simulink model "hydraulic_actuator"  (R2018a)
settings: Solver=ode23t  StartTime=0.0  StopTime=10.0  MaxStep=0.001  RelTol=1e-6  EnableMultiTasking=on
libraries: fl_lib x12, sh_lib x9, nesl_utility x4, simulink x1
Description:
  | Closed-Loop Electrohydraulic Actuator with Proportional Valve
  | 
  | This example shows an actuator that consists of a proportional 4-way directional valve
  | driving a double-acting hydraulic cylinder. The cylinder drives a load consisting of a mass,
  | viscous and Coulomb friction, constant force, and a spring. The actuator is powered
  | by a variable-displacement, pressure-compensated pump, driven by a constant velocity
  | motor. Pipelines between the valve, cylinder, pump, and the tank are simulated
  | with the Hydraulic Pipeline blocks.
  | 
  | 
  | Copyright 2008-2013 The MathWorks, Inc.
settings Model: ExtModeAutoUpdateStatusClock=off  Creator=MathWorks  LastModifiedBy=bpotter
settings DataIOCC: LimitDataPoints=on  SaveFormat=Array  SaveOutput=off  SignalLogging=off  DSMLogging=off  SaveTime=off
settings OptimizationCC: DefaultParameterBehavior=Inlined  ExpressionDepthLimit=2147483647  InitFltsAndDblsToZero=on  LifeSpan=inf
settings DebuggingCC: SaveWithParameterizedLinksMsg=none  SignalResolutionControl=TryResolveAllWithWarning  SolverPrmCheckMsg=warning  MultiTaskDSMMsg=warning  AllowSymbolicDim=off  StateNameClashWarn=warning  StrictBusMsg=ErrorOnBusTreatedAsVector  NonBusSignalsTreatedAsBus=error  SFUnexpectedBacktrackingDiag=warning  SFNoUnconditionalDefaultTransitionDiag=warning  SFExecutionAtInitializationDiag=none
settings HardwareCC: ProdBitPerPointer=32  ProdBitPerSizeT=32  ProdBitPerPtrDiffT=32  ProdLargestAtomicFloat=None  ProdEndianess=Unspecified  ProdWordSize=32  ProdHWDeviceType=32-bit Generic
settings ModelReferenceCC: PropagateSignalLabelsOutOfModel=off
settings CodeAppCC: StateflowObjectComments=on
settings GRTTargetCC: TargetFcnLib=ansi_tfl_tmw.mat  TargetLangStandard=C89/C90 (ANSI)  GeneratePreprocessorConditionals=Disable all  CombineOutputUpdateFcns=off  GRTInterface=on
settings ConfigComp: CovMetricSettings=dw  CovHtmlReporting=on  CovSaveCumulativeToWorkspaceVar=on  CovSaveSingleToWorkspaceVar=on  CovExternalEMLEnable=off  CovSFcnEnable=off
settings SimscapeCC: SimscapeNormalizeSystem=off

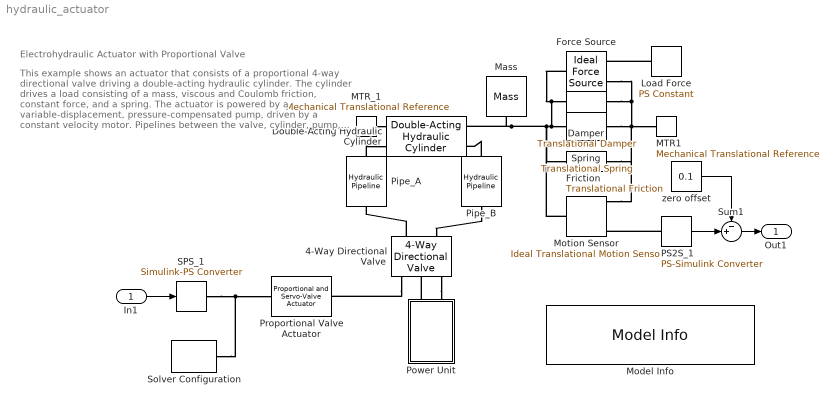
== system hydraulic_actuator ==
  note: This example shows an actuator that consists of a proportional
      | 4-way directional valve driving a double-acting hydraulic cylinder.
      | The cylinder drives a load consisting of a mass, viscous and
      | Coulomb friction, constant force, and a spring. The actuator is
      | powered by a variable-displacement, pressure-compensated pump,
      | driven by a constant velocity motor. Pipelines between the valve,
      | cylinder, pump, and the tank are simulated with the
      | Hydraulic Pipeline blocks.
  note: Electrohydraulic Actuator with Proportional Valve
  In1 : Inport  OutDataTypeStr=double  PortDimensions=1
  4-Way Directional Valve : sh_lib/Valves/Directional Valves/4-Way Directional Valve  Tag=Factory Generic  area_spec=1  mdl_type_identical=1  mdl_type_different=1  opening_max=0.01 m  area_max=0.00015 m^2  opening_max_P_A=0.005 m  area_max_P_A=0.5e-4 m^2  opening_max_P_B=0.005 m  area_max_P_B=0.5e-4 m^2  opening_max_A_T=0.005 m  area_max_A_T=0.5e-4 m^2  opening_max_B_T=0.005 m  area_max_B_T=0.5e-4 m^2  opening_area_tab=[-0.002 0 0.005 0.015] m  area_tab=[1e-12 4e-12 1e-05 1.02e-05] m^2  opening_flow_rate_tab=[-0.002 0 0.005 0.015] m  pressure_tab=[-5000000 -2000000 2000000 5000000] Pa  flow_rate_tab=[-1e-12 -6e-14 6000000000000 100000000000;-8e-08 -4e-08 4000000 8000000;-0.0025 -0.00103 0.001 0.0024;-0.00258 -0.001032 0.00106 0.00247] m^3/s  opening_area_tab_P_A=[-.002, 0, .002, .005, .015] m  area_tab_P_A=[1e-09, 2.0352e-07, 4.0736e-05, .00011438, .00034356] m^2  opening_flow_rate_tab_P_A=[-.002, 0, .002, .005, .015] m  pressure_tab_P_A=[-10000000, -5000000, -2000000, 2000000, 5000000, 10000000] Pa  flow_rate_tab_P_A=[-1e-07, -7.0711e-08, -4.4721e-08, 4.4721e-08, 7.0711e-08, 1e-07; -2.0352e-05, -1.4391e-05, -9.1017e-06, 9.1017e-06, 1.4391e-05, 2.0352e-05; -.0040736, -.0028805, -.0018218, .0018218, .0028805, .0040736; -.011438, -.0080879, -.0051152, .0051152, .0080879, .011438; -.034356, -.024293, -.015364, .015364, .024293, .034356] m^3/s  opening_area_tab_P_B=[-.002, 0, .002, .005, .015] m  area_tab_P_B=[1e-09, 2.0352e-07, 4.0736e-05, .00011438, .00034356] m^2  opening_flow_rate_tab_P_B=[-.002, 0, .002, .005, .015] m  pressure_tab_P_B=[-10000000, -5000000, -2000000, 2000000, 5000000, 10000000] Pa  flow_rate_tab_P_B=[-1e-07, -7.0711e-08, -4.4721e-08, 4.4721e-08, 7.0711e-08, 1e-07; -2.0352e-05, -1.4391e-05, -9.1017e-06, 9.1017e-06, 1.4391e-05, 2.0352e-05; -.0040736, -.0028805, -.0018218, .0018218, .0028805, .0040736; -.011438, -.0080879, -.0051152, .0051152, .0080879, .011438; -.034356, -.024293, -.015364, .015364, .024293, .034356] m^3/s  opening_area_tab_A_T=[-.002, 0, .002, .005, .015] m  area_tab_A_T=[1e-09, 2.0352e-07, 4.0736e-05, .00011438, .00034356] m^2  opening_flow_rate_tab_A_T=[-.002, 0, .002, .005, .015] m  pressure_tab_A_T=[-10000000, -5000000, -2000000, 2000000, 5000000, 10000000] Pa  flow_rate_tab_A_T=[-1e-07, -7.0711e-08, -4.4721e-08, 4.4721e-08, 7.0711e-08, 1e-07; -2.0352e-05, -1.4391e-05, -9.1017e-06, 9.1017e-06, 1.4391e-05, 2.0352e-05; -.0040736, -.0028805, -.0018218, .0018218, .0028805, .0040736; -.011438, -.0080879, -.0051152, .0051152, .0080879, .011438; -.034356, -.024293, -.015364, .015364, .024293, .034356] m^3/s  opening_area_tab_B_T=[-.002, 0, .002, .005, .015] m  area_tab_B_T=[1e-09, 2.0352e-07, 4.0736e-05, .00011438, .00034356] m^2  opening_flow_rate_tab_B_T=[-.002, 0, .002, .005, .015] m  pressure_tab_B_T=[-10000000, -5000000, -2000000, 2000000, 5000000, 10000000] Pa  flow_rate_tab_B_T=[-1e-07, -7.0711e-08, -4.4721e-08, 4.4721e-08, 7.0711e-08, 1e-07; -2.0352e-05, -1.4391e-05, -9.1017e-06, 9.1017e-06, 1.4391e-05, 2.0352e-05; -.0040736, -.0028805, -.0018218, .0018218, .0028805, .0040736; -.011438, -.0080879, -.0051152, .0051152, .0080879, .011438; -.034356, -.024293, -.015364, .015364, .024293, .034356] m^3/s  interp_method_identical=1  interp_method_different=1  extrap_method_identical=1  extrap_method_different=1  C_d=0.7  x_0_P_A=1e-05 m  x_0_P_B=1e-05 m  x_0_A_T=1e-05 m  x_0_B_T=1e-05 m  A_leak=1e-12 m^2  lam_spec=2  B_lam=0.999  Re_cr=12
      settings: SourceProductName=Simscape Fluids  SourceProductBaseCode=SH
  Damper : fl_lib/Mechanical/Translational Elements/Translational Damper  Tag=Factory Generic  D=2 s*N/m  v_specify=off  v_priority=High  v=0 m/s  v_nominal_specify=off  v_nominal_unit=m/s  v_nominal_value=1  f_specify=off  f_priority=High  f=0 N  f_nominal_specify=off  f_nominal_unit=N  f_nominal_value=1
  Double-Acting Hydraulic Cylinder : sh_lib/Hydraulic Cylinders/Double-Acting Hydraulic Cylinder  Tag=Factory Generic  area_A=0.004 m^2  area_B=0.002 m^2  stroke=0.2 m  init_pos=0.1 m  dead_vol_A=0.001 m^3  dead_vol_B=0.001 m^3  init_pressure_A=0 Pa  init_pressure_B=0 Pa  k_sh=1.4  stiff=1e+06 N/m  D=150 N/(m/s)  hardstop_model=3  transition=0.1 mm  or=1
      settings: SourceProductName=Simscape Fluids  SourceProductBaseCode=SH
  Force Source : fl_lib/Mechanical/Mechanical Sources/Ideal Force Source  Tag=Factory Generic
  Friction : fl_lib/Mechanical/Translational Elements/Translational Friction  Tag=Factory Generic  brkwy_frc=450 N  brkwy_vel=0.060623 m/s  Col_frc=450 N  visc_coef=0.01 s*N/m  v_specify=off  v_priority=High  v=0 m/s  v_nominal_specify=off  v_nominal_unit=m/s  v_nominal_value=1  f_specify=off  f_priority=High  f=0 N  f_nominal_specify=off  f_nominal_unit=N  f_nominal_value=1
      settings: SourceProductName=Simscape  SourceProductBaseCode=SS
  Load Force : fl_lib/Physical Signals/Sources/PS Constant  constant=-1000
  MTR1 : fl_lib/Mechanical/Translational Elements/Mechanical Translational Reference  Tag=Factory Generic
  MTR_1 : fl_lib/Mechanical/Translational Elements/Mechanical Translational Reference  Tag=Factory Generic
  Mass : fl_lib/Mechanical/Translational Elements/Mass  Tag=Factory Generic  mass=50 kg  v_specify=on  v_priority=High  v=0 m/s  v_nominal_specify=off  v_nominal_unit=m/s  v_nominal_value=1  f_specify=off  f_priority=High  f=0 N  f_nominal_specify=off  f_nominal_unit=N  f_nominal_value=1
  Model Info : simulink/Model-Wide Utilities/Model Info  Frame=on  DisplayStringWithTags=|  HorizontalTextAlignment=Center  LeftAlignmentValue=0.5
      | Model: %<ModelName>
      | Model Version: %<ModelVersion>
      | Last Modified: %<LastModificationDate>
      | 
      | Copyright 2016 The MathWorks, Inc.
  Motion Sensor : fl_lib/Mechanical/Mechanical Sensors/Ideal Translational Motion Sensor  Tag=Factory Generic  offset=0.1 m
  PS2S_1 : nesl_utility/PS-Simulink Converter  PhysicalDomain=network_engine_domain  SubClassName=ps_output  LeftPortType=input  RightPortType=output  PseudoPeriodic=off  Frequencies=[]  Unit=1  AffineConversion=off
  Pipe_A : sh_lib/Pipelines/Hydraulic Pipeline  Tag=Factory Generic  cs_type=1  d_in=0.02 m  area=0.0001 m^2  D_h=0.0112 m  s_factor=64  length=3 m  length_ad=2 m  roughness=1.5e-05 m  Re_lam=2000  Re_turb=4000  wall_type=1  pr_r_coef=2e-10 m/Pa  time_const=0.008 s  k_sh=1.4  initial_pressure=0 Pa
      settings: SourceProductName=Simscape Fluids  SourceProductBaseCode=SH
  Pipe_B : sh_lib/Pipelines/Hydraulic Pipeline  Tag=Factory Generic  cs_type=1  d_in=0.02 m  area=0.0001 m^2  D_h=0.0112 m  s_factor=64  length=3 m  length_ad=2 m  roughness=1.5e-05 m  Re_lam=2000  Re_turb=4000  wall_type=1  pr_r_coef=2e-10 m/Pa  time_const=0.008 s  k_sh=1.4  initial_pressure=0 Pa
      settings: SourceProductName=Simscape Fluids  SourceProductBaseCode=SH
  Power Unit : Subsystem
  Proportional Valve Actuator : sh_lib/Valves/Valve Actuators/Proportional and Servo-Valve Actuator  Tag=Factory Generic  gain=250  time_constant=0.002 s  saturation=0.3
      settings: SourceProductName=Simscape Fluids  SourceProductBaseCode=SH
  SPS_1 : nesl_utility/Simulink-PS Converter  PhysicalDomain=network_engine_domain  SubClassName=ps_input  LeftPortType=input  RightPortType=output  PseudoPeriodic=off  Frequencies=[]  NoiseDistribution=none  NoiseParameters=[]  Unit=1  AffineConversion=off  FilteringAndDerivatives=zero  SimscapeFilterOrder=1  InputFilterTimeConstant=.001  UdotUserProvided=0
  Solver Configuration : nesl_utility/Solver Configuration  PhysicalDomain=network_engine_domain  SubClassName=solver  LeftPortType=input  RightPortType=generic  Tones=[]  Harmonics=[]  SimulateNoise=off  Profile=off  UseLocalSampling=off  EnableSwitchedLinearOptims=on  FrequencyDomain=off  UseCCode=off  RelTol=0.001  AbsTol=1e-06  MinStep=1e-09  ToWorkspace=off  RevertToSquareIcSolve=off  NumHomotopyIterations=100  PhasorMode=off  PhasorModeNumHarmonics=1  DoDC=off  ResidualTolerance=1e-9  UseLocalSolver=off  LocalSolverChoice=NE_BACKWARD_EULER_ADVANCER  LocalSolverSampleTime=.001  DoFixedCost=off  MaxNonlinIter=3  MaxModeIter=2  LinearAlgebra=Sparse  EquationFormulation=NE_TIME_EF  DelaysMemoryBudget=1024  AutomaticFiltering=on  FilteringTimeConstant=0.001
  Spring : fl_lib/Mechanical/Translational Elements/Translational Spring  Tag=Factory Generic  spr_rate=15000 N/m  v_specify=off  v_priority=High  v=0 m/s  v_nominal_specify=off  v_nominal_unit=m/s  v_nominal_value=1  f_specify=off  f_priority=High  f=0 N  f_nominal_specify=off  f_nominal_unit=N  f_nominal_value=1  x_specify=on  x_priority=High  x=0 m  x_nominal_specify=off  x_nominal_unit=m  x_nominal_value=1
  Sum1 : Sum  Inputs=-+|
  zero offset : Constant  Value=0.1
  Out1 : Outport  OutDataTypeStr=double  PortDimensions=1
  wires:
  In1/1 -> SPS_1/1
  Sum1/1 -> Out1/1
  PS2S_1/1 -> Sum1/2
  zero offset/1 -> Sum1/1
  connections:
  MTR_1/LConn1 -- Double-Acting Hydraulic Cylinder/LConn1
  Damper/LConn1 -- Motion Sensor/LConn1 -- Friction/LConn1 -- Spring/LConn1 -- Mass/LConn1 -- Double-Acting Hydraulic Cylinder/RConn1 -- Force Source/LConn1
  4-Way Directional Valve/LConn1 -- Pipe_A/LConn1
  Pipe_B/LConn1 -- Double-Acting Hydraulic Cylinder/RConn2
  Pipe_B/RConn1 -- 4-Way Directional Valve/LConn2
  4-Way Directional Valve/RConn3 -- Power Unit/RConn2
  4-Way Directional Valve/RConn1 -- Proportional Valve Actuator/RConn1
  SPS_1/RConn1 -- Solver Configuration/RConn1 -- Proportional Valve Actuator/LConn1
  Power Unit/RConn1 -- 4-Way Directional Valve/RConn2
  Pipe_A/RConn1 -- Double-Acting Hydraulic Cylinder/LConn2
  Load Force/RConn1 -- Force Source/RConn1
  Damper/RConn1 -- Motion Sensor/RConn1 -- Friction/RConn1 -- Spring/RConn1 -- MTR1/LConn1 -- Force Source/RConn2
  PS2S_1/LConn1 -- Motion Sensor/RConn3

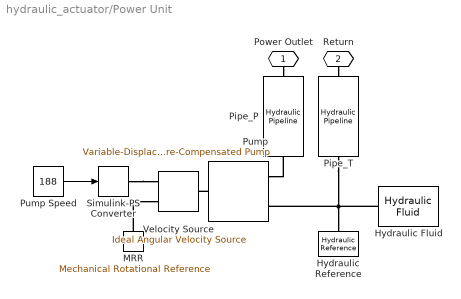
== system hydraulic_actuator/Power Unit ==
  Hydraulic Reference : fl_lib/Hydraulic/Hydraulic Elements/Hydraulic Reference  Tag=Factory Generic
      settings: SourceProductName=Simscape
  Hydraulic Fluid : sh_lib/Hydraulic Utilities/Hydraulic Fluid  Tag=Factory Generic  DataSource=1  SelFluid=2  SysTemp=60  TrapAir=0.001  ViscDerFactor=1  range_error=2
      settings: SourceProductName=Simscape Fluids
  MRR : fl_lib/Mechanical/Rotational Elements/Mechanical Rotational Reference  Tag=Factory Generic
  Pipe_P : sh_lib/Pipelines/Hydraulic Pipeline  Tag=Factory Generic  cs_type=1  d_in=0.02 m  area=0.0001 m^2  D_h=0.0112 m  s_factor=64  length=6 m  length_ad=3 m  roughness=1.5e-05 m  Re_lam=2000  Re_turb=4000  wall_type=1  pr_r_coef=2e-10 m/Pa  time_const=0.008 s  k_sh=1.4  initial_pressure=0 Pa
      settings: SourceProductName=Simscape Fluids  SourceProductBaseCode=SH
  Pipe_T : sh_lib/Pipelines/Hydraulic Pipeline  Tag=Factory Generic  cs_type=1  d_in=0.02 m  area=0.0001 m^2  D_h=0.0112 m  s_factor=64  length=6 m  length_ad=2 m  roughness=1.5e-05 m  Re_lam=2000  Re_turb=4000  wall_type=1  pr_r_coef=2e-10 m/Pa  time_const=0.008 s  k_sh=1.4  initial_pressure=0 Pa
      settings: SourceProductName=Simscape Fluids  SourceProductBaseCode=SH
  Pump : sh_lib/Pumps and Motors/Variable-Displacement Pressure-Compensated Pump  Tag=Factory Generic  D_max=5e-06 m^3/rad  pr_set=6.0e+06 Pa  pr_reg=600000 Pa  efficiency_vol=0.9  efficiency_tot=0.75  pr_nominal=1e+07 Pa  w_nominal=188 rad/s  visc_nominal=18 cSt  dens_nominal=950 kg/m^3
      settings: SourceProductName=Simscape Fluids  SourceProductBaseCode=SH
  Pump Speed : Constant  Value=188
  Simulink-PS Converter : nesl_utility/Simulink-PS Converter  PhysicalDomain=network_engine_domain  SubClassName=ps_input  LeftPortType=input  RightPortType=output  PseudoPeriodic=off  Frequencies=[]  NoiseDistribution=none  NoiseParameters=[]  Unit=1  AffineConversion=off  FilteringAndDerivatives=zero  SimscapeFilterOrder=1  InputFilterTimeConstant=.001  UdotUserProvided=0
  Velocity Source : fl_lib/Mechanical/Mechanical Sources/Ideal Angular Velocity Source  Tag=Factory Generic
  Power Outlet : PMIOPort  Side=Right
  Return : PMIOPort  Port=2  Side=Right
  wires:
  Pump Speed/1 -> Simulink-PS Converter/1
  connections:
  Pump/RConn1 -- Pipe_P/LConn1
  Pipe_T/RConn1 -- Hydraulic Fluid/RConn1 -- Pump/RConn2 -- Hydraulic Reference/LConn1
  MRR/LConn1 -- Velocity Source/RConn2
  Simulink-PS Converter/RConn1 -- Velocity Source/RConn1
  Pump/LConn1 -- Velocity Source/LConn1
  Power Outlet/RConn1 -- Pipe_P/RConn1
  Return/RConn1 -- Pipe_T/LConn1
